simulink model "translation"  (R2020a)
settings: Solver=VariableStepAuto  StartTime=0.0  StopTime=1000  RelTol=1e-3
values from neighbouring files (symbols this model uses):
  euler_angles_NfromB_0_deg = [0; 0; 0]    [p1partApartI.m]
  EvB_BfromE_mps = [150; 0; 0]    [p1partApartI.m]
  ExE_BfromE_0_m = [re_m; 0; 0]    [p1partApartI.m]
  ll_NfromE_deg = [0, 0]    [p1partApartI.m]
libraries: coordinate_transforms x5, aerolibutil x2
settings Model: Creator=Nikita  LastModifiedBy=Nikita

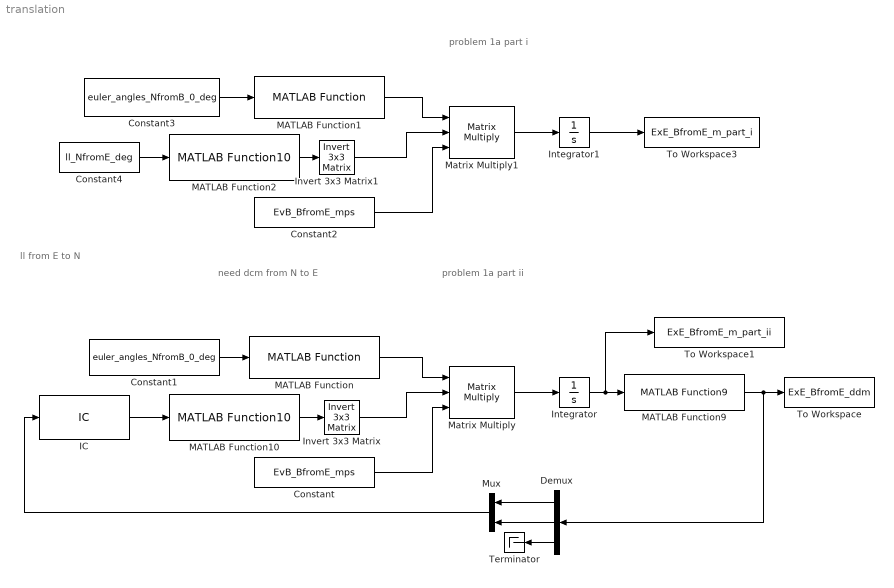
== system translation ==
  note: need dcm from N to E
  note: ll from E to N
  note: problem 1a part ii
  note: problem 1a part i
  Constant : Constant  Value=EvB_BfromE_mps
  Constant1 : Constant  Value=euler_angles_NfromB_0_deg
  Constant2 : Constant  Value=EvB_BfromE_mps
  Constant3 : Constant  Value=euler_angles_NfromB_0_deg
  Constant4 : Constant  Value=ll_NfromE_deg
  Demux : Demux  Outputs=3
  IC : InitialCondition  Value=ll_NfromE_deg
  Integrator : Integrator  InitialCondition=ExE_BfromE_0_m
  Integrator1 : Integrator  InitialCondition=ExE_BfromE_0_m
  Invert 3x3 Matrix : aerolibutil/Invert  3x3 Matrix
  Invert 3x3 Matrix1 : aerolibutil/Invert  3x3 Matrix
  MATLAB Function : coordinate_transforms/MATLAB Function  SystemSampleTime=-1  Latency=0  AutoFrameSizeCalculation=off
  MATLAB Function1 : coordinate_transforms/MATLAB Function  SystemSampleTime=-1  Latency=0  AutoFrameSizeCalculation=off
  MATLAB Function10 : coordinate_transforms/MATLAB Function10  SystemSampleTime=-1  Latency=0  AutoFrameSizeCalculation=off
  MATLAB Function2 : coordinate_transforms/MATLAB Function10  SystemSampleTime=-1  Latency=0  AutoFrameSizeCalculation=off
  MATLAB Function9 : coordinate_transforms/MATLAB Function9  SystemSampleTime=-1  Latency=0  AutoFrameSizeCalculation=off
  Matrix Multiply : Product  Inputs=3  Multiplication=Matrix(*)
  Matrix Multiply1 : Product  Inputs=3  Multiplication=Matrix(*)
  Mux : Mux  Inputs=2
  Terminator : Terminator
  To Workspace : ToWorkspace  VariableName=ExE_BfromE_ddm  SampleTime=-1
  To Workspace1 : ToWorkspace  VariableName=ExE_BfromE_m_part_ii  SampleTime=-1
  To Workspace3 : ToWorkspace  VariableName=ExE_BfromE_m_part_i  SampleTime=-1
  wires:
  MATLAB Function/1 -> Matrix Multiply/1
  Constant1/1 -> MATLAB Function/1
  Constant/1 -> Matrix Multiply/3
  Matrix Multiply/1 -> Integrator/1
  Integrator/1 -> To Workspace1/1, MATLAB Function9/1
  MATLAB Function9/1 -> Demux/1, To Workspace/1
  IC/1 -> MATLAB Function10/1
  MATLAB Function10/1 -> Invert 3x3 Matrix/1
  Mux/1 -> IC/1
  Demux/1 -> Mux/1
  Demux/2 -> Mux/2
  Demux/3 -> Terminator/1
  Constant4/1 -> MATLAB Function2/1
  Integrator1/1 -> To Workspace3/1
  MATLAB Function2/1 -> Invert 3x3 Matrix1/1
  Constant3/1 -> MATLAB Function1/1
  MATLAB Function1/1 -> Matrix Multiply1/1
  Matrix Multiply1/1 -> Integrator1/1
  Constant2/1 -> Matrix Multiply1/3
  Invert 3x3 Matrix1/1 -> Matrix Multiply1/2
  Invert 3x3 Matrix/1 -> Matrix Multiply/2
